simulink model "cstr_sim1"  (R2017a)
settings: Solver=ode45  StartTime=0  StopTime=24  RelTol=1e-3  AbsTol=1e-6  EnableMultiTasking=on
libraries: slident x3
settings Model: Creator=The MathWorks, Inc.  LastModifiedBy=ljxia_000
settings DataIOCC: LimitDataPoints=on  SaveFormat=Array
settings OptimizationCC: InitFltsAndDblsToZero=on  LifeSpan=inf
settings DebuggingCC: SaveWithParameterizedLinksMsg=none  UnderspecifiedInitializationDetection=Classic  MergeDetectMultiDrivingBlocksExec=none  SignalResolutionControl=TryResolveAllWithWarning  SolverPrmCheckMsg=warning  FcnCallInpInsideContextMsg=warning  StateNameClashWarn=warning  StrictBusMsg=Warning  SFUnexpectedBacktrackingDiag=warning  SFNoUnconditionalDefaultTransitionDiag=warning  SFExecutionAtInitializationDiag=none
settings HardwareCC: ProdBitPerPointer=32  ProdBitPerSizeT=32  ProdBitPerPtrDiffT=32  ProdLargestAtomicFloat=None  ProdIntDivRoundTo=Undefined  ProdEndianess=Unspecified  ProdWordSize=32  ProdHWDeviceType=32-bit Generic
settings ModelReferenceCC: PropagateSignalLabelsOutOfModel=off
settings GRTTargetCC: TargetFcnLib=ansi_tfl_tmw.mat  TargetLangStandard=C89/C90 (ANSI)  CombineOutputUpdateFcns=off  GRTInterface=on
settings ConfigComp: CovMetricSettings=dw  CovHtmlReporting=on  CovSaveCumulativeToWorkspaceVar=on  CovSaveSingleToWorkspaceVar=on  CovExternalEMLEnable=off

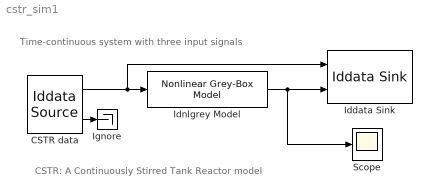
== system cstr_sim1 ==
  note: Time-continuous system with three input signals
  note: CSTR: A Continuously Stirred Tank Reactor model
  CSTR data : slident/Iddata Source  iddataobj=zv
      settings: SourceProductName=System Identification Toolbox  SourceProductBaseCode=ID
  Iddata Sink : slident/Iddata Sink  datasetname=zsim  Ts=0.1  isu=off  isy=off
      settings: SourceProductName=System Identification Toolbox  SourceProductBaseCode=ID
  Idnlgrey Model : slident/Models/Nonlinear Grey-Box Model  nlsys=nlgr  X0='m'
      settings: SourceProductName=System Identification Toolbox  SourceProductBaseCode=ID
  Ignore : Terminator
  Scope : Scope
  wires:
  CSTR data/2 -> Ignore/1
  Idnlgrey Model/1 -> Iddata Sink/2, Scope/1
  CSTR data/1 -> Iddata Sink/1, Idnlgrey Model/1
